simulink model "BDamperError"  (R2018b)
settings: Solver=FixedStepAuto  StartTime=0.0  StopTime=10.0  RelTol=1e-3
undefined symbols (not defined in the file): VDamperErrorHigh, VDamperErrorLow
libraries: simulink x8
settings Model: DataDictionary=Master_Dictionary.sldd  Creator=torni  LastModifiedBy=oxbro
settings RTWCC: SystemTargetFile=irt.tlc  TemplateMakefile=irt_default_tmf  Description=INTECRIO Real-Time Target
settings STFCustomTargetCC: TargetLangStandard=C99 (ISO)  CombineOutputUpdateFcns=on  MatFileLogging=on  SystemTargetFile=irt.tlc
settings GRTTargetCC: ParMdlRefBuildCompliant=off  CompOptLevelCompliant=off  ConcurrentExecutionCompliant=off  CPPClassGenCompliant=off  UseToolchainInfoCompliant=off

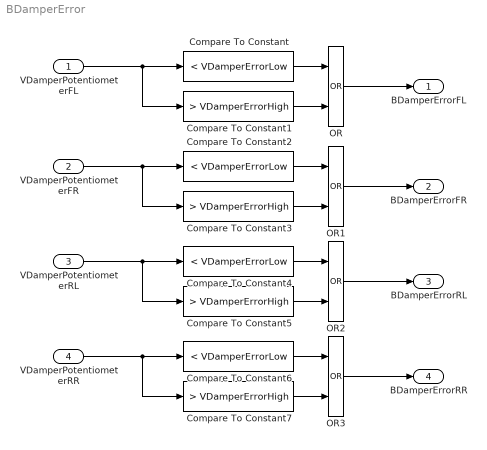
== system BDamperError ==
  VDamperPotentiometerFL : Inport  OutDataTypeStr=double
  "VDamperPotentiometerFR " : Inport  Port=2  OutDataTypeStr=double
  VDamperPotentiometerRL : Inport  Port=3  OutDataTypeStr=double
  VDamperPotentiometerRR : Inport  Port=4  OutDataTypeStr=double
  Compare To Constant{,2,4,6} (4 alike) : simulink/Logic and Bit Operations/Compare To Constant  relop=<  const=VDamperErrorLow  OutDataTypeStr=boolean
  Compare To Constant{1,3,5,7} (4 alike) : simulink/Logic and Bit Operations/Compare To Constant  relop=>  const=VDamperErrorHigh  OutDataTypeStr=boolean
  OR{,1..3} (4 alike) : Logic  Operator=OR  AllPortsSameDT=off  OutDataTypeStr=boolean
  BDamperErrorFL : Outport  OutDataTypeStr=boolean
  BDamperErrorFR : Outport  Port=2  OutDataTypeStr=boolean
  BDamperErrorRL : Outport  Port=3  OutDataTypeStr=boolean
  BDamperErrorRR : Outport  Port=4  OutDataTypeStr=boolean
  wires:
  Compare To Constant1/1 -> OR/2
  Compare To Constant/1 -> OR/1
  OR3/1 -> BDamperErrorRR/1
  VDamperPotentiometerFL/1 -> Compare To Constant1/1, Compare To Constant/1
  OR/1 -> BDamperErrorFL/1
  OR1/1 -> BDamperErrorFR/1
  "VDamperPotentiometerFR "/1 -> Compare To Constant2/1, Compare To Constant3/1
  Compare To Constant2/1 -> OR1/1
  Compare To Constant3/1 -> OR1/2
  Compare To Constant5/1 -> OR2/2
  Compare To Constant4/1 -> OR2/1
  VDamperPotentiometerRL/1 -> Compare To Constant5/1, Compare To Constant4/1
  OR2/1 -> BDamperErrorRL/1
  VDamperPotentiometerRR/1 -> Compare To Constant6/1, Compare To Constant7/1
  Compare To Constant6/1 -> OR3/1
  Compare To Constant7/1 -> OR3/2
